simulink model "t7_videoclase3_masa_resorte_amortiguador_v2"  (R2022b)
settings: Solver=ode4  StartTime=0.0  StopTime=20  FixedStep=0.01  MaxStep=1.0  RelTol=1e-3
model workspace (MATLAB code in the model file):
  | % número de simulaciones
  | n = 1000;
  | 
  | % parámetros
  | m = 3;
  | s = .1;
  | 
  | c1 = 0.1;
  | c2 = 0.3;
  | 
  | k1 = 2;
  | k2 = 3;
settings Model: Creator=jibmo  LastModifiedBy=scpmoxxa
settings DataIOCC: SaveFormat=Array  SaveState=on

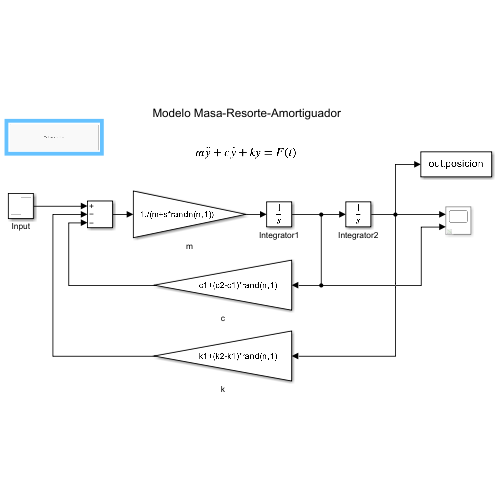
[thumbnail: Simulink's stored preview of the top-level diagram]
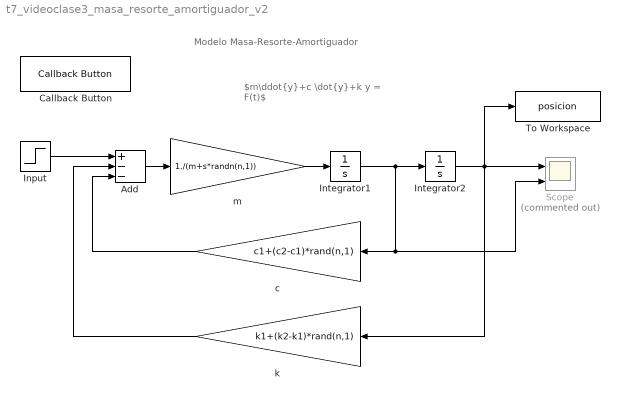
== system t7_videoclase3_masa_resorte_amortiguador_v2 ==
  note: Modelo Masa-Resorte-Amortiguador
  note: $m\ddot{y}+c \dot{y}+k y = F(t)$
  Add : Sum  Inputs=+--
  Callback Button : CallbackButton
      settings: ClickFcn=|
      | close all
      | 
      | position = out.posicion(end,:);
      | % Análisis de los resultados
      | mean_displacement = mean(position);
      | std_displacement = std(position);
      | 
      | % Visualization of the results
      | figure;
      | bins = 128;
      | h = histogram(position, bins, 'Normalization', 'pdf'); % Normalize the histogram to get a probability density
      | title('Final Displacement Distribution', 'Interpreter', 'none');
      | xlabel('Displacement', 'Interpreter', 'none');
      | ylabel('Probability Density', 'Interpreter', 'none');
      | 
      | % Fit a normal distribution
      | x_values = linspace(min(position), max(position), 100);
      | pdf_normal = normpdf(x_values, mean_displacement, std_displacement);
      | 
      | % Add the fitted normal distribution curve
      | hold on;
      | plot(x_values, pdf_normal, 'b-', 'LineWidth', 2, 'DisplayName', 'Normal Distribution');
      | 
      | % Add lines for the mean and standard deviation
      | yLimits = ylim; % Get the current y-axis limits
      | plot([mean_displacement, mean_displacement], yLimits, 'r--', 'LineWidth', 2, 'DisplayName', 'Mean');
      | plot([mean_displacement - std_displacement, mean_displacement - std_displacement], yLimits, 'g--', 'LineWidth', 2, 'DisplayName', 'Standard Deviation (-)');
      | plot([mean_displacement + std_displacement, mean_displacement + std_displacement], yLimits, 'g--', 'LineWidth', 2, 'DisplayName', 'Standard Deviation (+)');
      | 
      | % Add legend
      | legend('show', 'Interpreter', 'none');
      | 
      | % Display mean and standard deviation values in the title
      | title(sprintf('Final Displacement Distribution\nMean = %.2f, Standard Deviation = %.2f', mean_displacement, std_displacement), 'Interpreter', 'none');
      | hold off;
      | 
      | % Adjust global font properties to ensure proper display of special characters
      | set(gca, 'FontName', 'Arial', 'FontSize', 12);
  Input : Step  SampleTime=0
  Integrator1 : Integrator
  Integrator2 : Integrator  InitialCondition=0.1+(.5-0.1)*rand
  Scope : Scope  Commented=on  NumInputPorts=2
  To Workspace : ToWorkspace  VariableName=posicion  SampleTime=-1
  c : Gain  SCDEnableBlockLinearizationSpecification=on  Gain=c1+(c2-c1)*rand(n,1)
  k : Gain  SCDEnableBlockLinearizationSpecification=on  Gain=k1+(k2-k1)*rand(n,1)
  m : Gain  SCDEnableBlockLinearizationSpecification=on  Gain=1./(m+s*randn(n,1))
  wires:
  m/1 -> Integrator1/1
  Integrator1/1 -> c/1, Scope/2, Integrator2/1
  Integrator2/1 -> To Workspace/1, k/1, Scope/1
  Add/1 -> m/1
  c/1 -> Add/3
  k/1 -> Add/2
  Input/1 -> Add/1
